simulink model "MPCView2D"  (R2025b)
settings: Solver=VariableStepAuto  StartTime=0.0  StopTime=25  RelTol=1e-3
values from neighbouring files (symbols this model uses):
  sys_c = ss(A, B, C, D,      'StateName',  {'Angulo (rad)', 'Velocidad (rad/s)'},      'InputName',  {'Torque (Nm)'},      'OutputName', {'Angulo (rad)'})    [Modelo.m]
libraries: simulink x2, mpclib x1
settings Model: Creator=Camilo  LastModifiedBy=Camilo

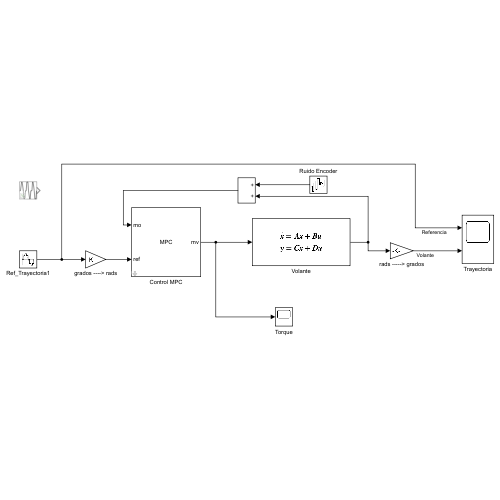
[thumbnail: Simulink's stored preview of the top-level diagram]
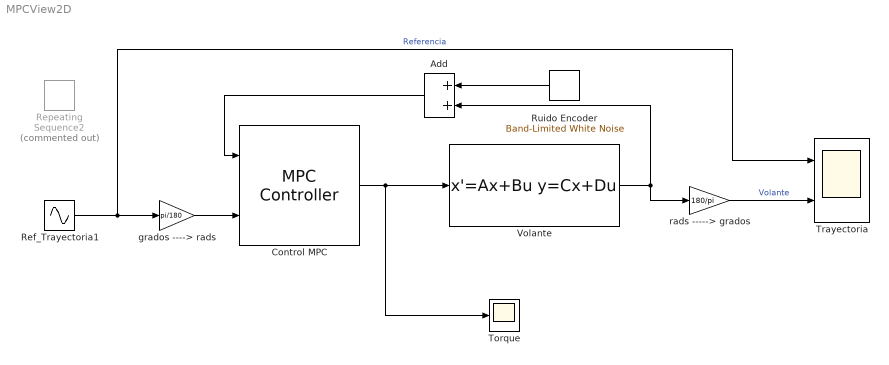
== system MPCView2D ==
  Add : Sum
  Control MPC : mpclib/MPC Controller  SCDEnableBlockLinearizationSpecification=on  mpcobj=mpc1  is_multiple=0  enable_value=0  return_u0=off  updateMPCinCallerWorkspace=on  md_inport=off  mv_inport=off  uref_inport=off  return_cost=off  return_mvseq=off  return_qpstatus=off  return_xseq=off  return_state=off  return_ovseq=off  state_inport=off  umin_inport=off  umax_inport=off  ymin_inport=off  ymax_inport=off  cc_inport=off  ywt_inport=off  uwt_inport=off  duwt_inport=off  rhoeps_inport=off  pm_inport=off  MaximumP=10  HorizonChoice=FixedHorizon  n_ts=0.05  n_p=10  n_mv=1  n_md=0  n_ud=0  n_mo=1  n_uo=0  BlockDataType=double  SampleTimeInherited=off  switch_inport=off
  Ref_Trayectoria1 : Sin  Amplitude=180  Frequency=0.3  SampleTime=0.01
  Repeating Sequence2 : simulink/Sources/Repeating Sequence  Commented=on  rep_seq_t=[0, 2, 4, 6, 8, 10, 12, 14]  rep_seq_y=[0, 0, 90, 90, 0, -90, -90, 0]
  Ruido Encoder : simulink/Sources/Band-Limited White Noise  Cov=0.000001  Ts=0.01  seed=[23341]
  Torque : Scope
      settings: ActiveDisplayYMinimum=-0.20883858224071286  ActiveDisplayYMaximum=0.64568253382188179
  Trayectoria : Scope  NumInputPorts=2
      settings: ActiveDisplayYMinimum=-224.99994589949767  ActiveDisplayYMaximum=224.99984910593238
  Volante : StateSpace  A=sys_c.A  B=sys_c.B  C=sys_c.C  D=sys_c.D  InitialCondition=[0;0]
  grados ----> rads : Gain  Gain=pi/180
  rads -----> grados : Gain  Gain=180/pi
  wires:
  Control MPC/1 -> Torque/1, Volante/1
  Volante/1 -> rads -----> grados/1, Add/2
  Ruido Encoder/1 -> Add/1
  Add/1 -> Control MPC/1
  grados ----> rads/1 -> Control MPC/2
  Ref_Trayectoria1/1 -> Trayectoria/1, grados ----> rads/1  "Referencia"
  rads -----> grados/1 -> Trayectoria/2  "Volante"
